simulink model "Lab13remix"  (R2025b)
settings: Solver=VariableStepAuto  StartTime=0.0  StopTime=30  RelTol=1e-3
values from neighbouring files (symbols this model uses):
  CDdatum = CD(1:47,2)    [Presimulink.m]
  CLdatum = CL(1:47,2)    [Presimulink.m]
  Cmdatum = Cm(1:47,2)    [Presimulink.m]
  dCDelev = [dCDn10 dCDn5 dCD0 dCDp5 dCDp10]    [Presimulink.m]
  dCLelev = [dCLn10 dCLn5 dCL0 dCLp5 dCLp10]    [Presimulink.m]
  dCmelev = [dCmn10 dCmn5 dCm0 dCmp5 dCmp10]    [Presimulink.m]
undefined symbols (not defined in the file or in its folder): Cn_datum, Croll_datum, CY_datum, dCn_aileron, dCn_rudder, dCroll_aileron, dCroll_rudder, dCY_aileron, dCY_rudder
libraries: aerolibadyn x1, aerolibasang x1, aerolibanim x1
settings Model: Creator=andyf  LastModifiedBy=andyf

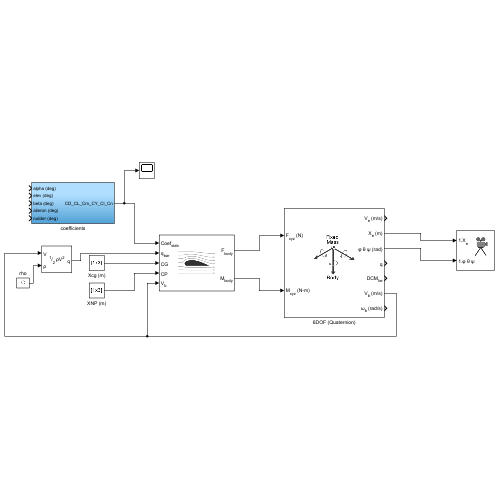
[thumbnail: Simulink's stored preview of the top-level diagram]
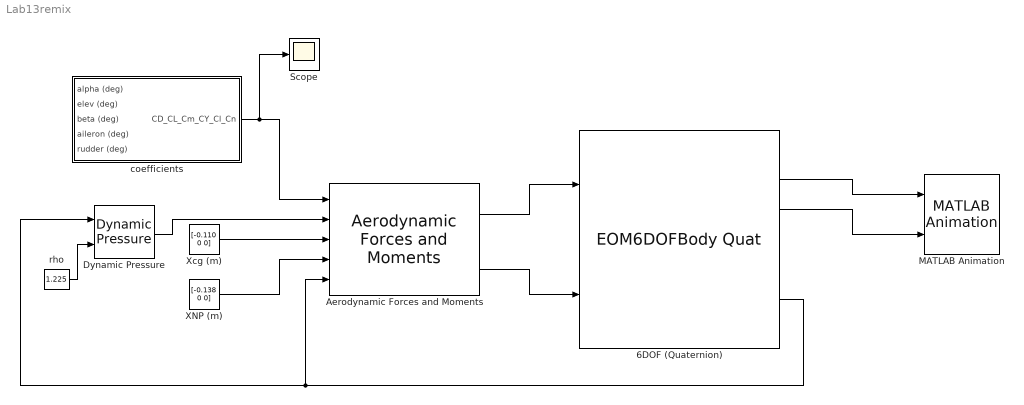
== system Lab13remix ==
  6DOF (Quaternion) : EOM6DOFBodyQuat  xme_0=[0 0 -200]  Vm_0=[15 0 2.5]  eul_0=[0 1.4*pi/180 0]  mass_0=0.45
  "Aerodynamic Forces and Moments " : aerolibadyn/Aerodynamic Forces and Moments   inputAxes=Stability  outputForceAxes=Body  outputMomentAxes=Body  S=0.15  b=1  cbar=0.156
  Dynamic Pressure : aerolibasang/Dynamic Pressure
  MATLAB Animation : aerolibanim/MATLAB Animation  Tag=Matlab Animation 6 DOF  Vehicles=1  Geometries='astredwedge.mat'  BoundingBoxCoordinates=[-50,50,-50,50,-50,50]  CameraOffset=[-150,-50,0]  CameraViewAngle=3  SampleTime=0.2  FigurePosition=[8.014000e+02,208,4.480000e+02,450]
  Scope : Scope
      settings: ActiveDisplayYMinimum=-0.18143250188090621  ActiveDisplayYMaximum=0.139826593948562
  XNP (m) : Constant  Value=[-0.138 0 0]
  Xcg (m) : Constant  Value=[-0.110 0 0]
  coefficients : Subsystem
  rho : Constant  Value=1.225
  wires:
  coefficients/1(CD_CL_Cm_CY_Cl_Cn) -> Scope/1, "Aerodynamic Forces and Moments "/1
  Xcg (m)/1 -> "Aerodynamic Forces and Moments "/3
  XNP (m)/1 -> "Aerodynamic Forces and Moments "/4
  "Aerodynamic Forces and Moments "/1 -> 6DOF (Quaternion)/1
  "Aerodynamic Forces and Moments "/2 -> 6DOF (Quaternion)/2
  rho/1 -> Dynamic Pressure/2
  6DOF (Quaternion)/6 -> Dynamic Pressure/1, "Aerodynamic Forces and Moments "/5
  Dynamic Pressure/1 -> "Aerodynamic Forces and Moments "/2
  6DOF (Quaternion)/3 -> MATLAB Animation/2
  6DOF (Quaternion)/2 -> MATLAB Animation/1

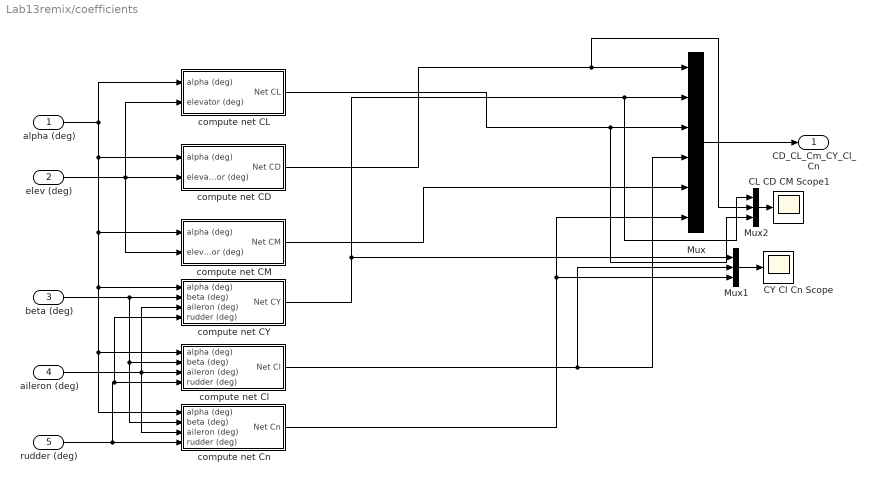
== system Lab13remix/coefficients ==
  alpha (deg) : Inport
  elev (deg) : Inport  Port=2
  beta (deg) : Inport  Port=3
  aileron (deg) : Inport  Port=4
  rudder (deg) : Inport  Port=5
  CL CD CM Scope1 : Scope
      settings: ActiveDisplayYMinimum=-5.92708  ActiveDisplayYMaximum=4.2418  DataLoggingVariableName=ScopeData4
  CY Cl Cn Scope : Scope
      settings: ActiveDisplayYMinimum=-0.00278  ActiveDisplayYMaximum=0.00326  DataLoggingVariableName=ScopeData3
  Mux : Mux  Inputs=6
  Mux1 : Mux  Inputs=3
  Mux2 : Mux  Inputs=3
  compute net CD : Subsystem
  compute net CL : Subsystem
  compute net CM : Subsystem
  compute net CY : Subsystem
  compute net Cl : Subsystem
  compute net Cn : Subsystem
  CD_CL_Cm_CY_Cl_Cn : Outport  VectorParamsAs1DForOutWhenUnconnected=off
  wires:
  compute net Cn/1(Net Cn) -> Mux1/3, Mux/6
  Mux/1 -> CD_CL_Cm_CY_Cl_Cn/1
  elev (deg)/1 -> compute net CD/2(elevator (deg)), compute net CM/2(elevator (deg)), compute net CL/2(elevator (deg))
  alpha (deg)/1 -> compute net CD/1(alpha (deg)), compute net Cn/1(alpha (deg)), compute net Cl/1(alpha (deg)), compute net CY/1(alpha (deg)), compute net CM/1(alpha (deg)), compute net CL/1(alpha (deg))
  compute net CD/1(Net CD) -> Mux2/2, Mux/1
  compute net CL/1(Net CL) -> Mux2/3, Mux/3
  compute net CM/1(Net CM) -> Mux/5
  compute net Cl/1(Net Cl) -> Mux1/2, Mux/4
  compute net CY/1(Net CY) -> Mux1/1, Mux2/1, Mux/2
  aileron (deg)/1 -> compute net Cl/3(aileron (deg)), compute net CY/3(aileron (deg)), compute net Cn/3(aileron (deg))
  beta (deg)/1 -> compute net Cn/2(beta (deg)), compute net Cl/2(beta (deg)), compute net CY/2(beta (deg))
  rudder (deg)/1 -> compute net CY/4(rudder (deg)), compute net Cl/4(rudder (deg)), compute net Cn/4(rudder (deg))
  Mux1/1 -> CY Cl Cn Scope/1
  Mux2/1 -> CL CD CM Scope1/1

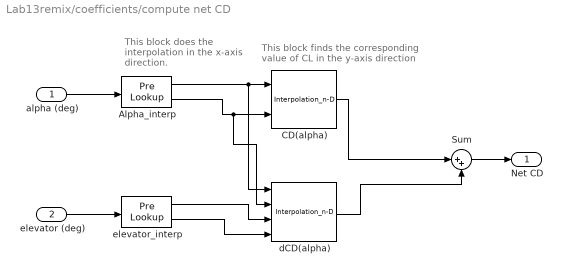
== system Lab13remix/coefficients/compute net CD ==
  note: This block finds the corresponding
      | value of CL in the y-axis direction
  note: This block does the interpolation in the
      | x-axis direction.
  alpha (deg) : Inport
  elevator (deg) : Inport  Port=2
  Alpha_interp : PreLookup  BreakpointsData=alpha  BeginIndexSearchUsingPreviousIndexResult=on  ExtrapMethod=Linear
  CD(alpha) : Interpolation_n-D  NumberOfTableDimensions=1  Table=CDdatum  RemoveProtectionIndex=on
      settings: InputPortMap=u0,u1
  Sum : Sum  Inputs=|++
  dCD(alpha) : Interpolation_n-D  Table=dCDelev
  elevator_interp : PreLookup  BreakpointsData=delev  BeginIndexSearchUsingPreviousIndexResult=on  ExtrapMethod=Linear
  Net CD : Outport  VectorParamsAs1DForOutWhenUnconnected=off
  wires:
  Alpha_interp/1 -> dCD(alpha)/1, CD(alpha)/1
  Alpha_interp/2 -> dCD(alpha)/2, CD(alpha)/2
  CD(alpha)/1 -> Sum/1
  alpha (deg)/1 -> Alpha_interp/1
  elevator (deg)/1 -> elevator_interp/1
  elevator_interp/2 -> dCD(alpha)/4
  elevator_interp/1 -> dCD(alpha)/3
  dCD(alpha)/1 -> Sum/2
  Sum/1 -> Net CD/1

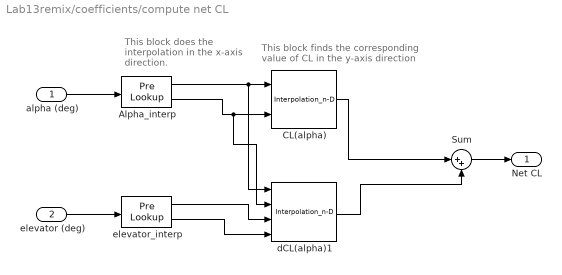
== system Lab13remix/coefficients/compute net CL ==
  note: This block finds the corresponding
      | value of CL in the y-axis direction
  note: This block does the interpolation in the
      | x-axis direction.
  alpha (deg) : Inport
  elevator (deg) : Inport  Port=2
  Alpha_interp : PreLookup  BreakpointsData=alpha  BeginIndexSearchUsingPreviousIndexResult=on  ExtrapMethod=Linear
  CL(alpha) : Interpolation_n-D  NumberOfTableDimensions=1  Table=CLdatum  RemoveProtectionIndex=on
      settings: InputPortMap=u0,u1
  Sum : Sum  Inputs=|++
  dCL(alpha)1 : Interpolation_n-D  Table=dCLelev
  elevator_interp : PreLookup  BreakpointsData=delev  BeginIndexSearchUsingPreviousIndexResult=on  ExtrapMethod=Linear
  Net CL : Outport  VectorParamsAs1DForOutWhenUnconnected=off
  wires:
  Alpha_interp/1 -> dCL(alpha)1/1, CL(alpha)/1
  Alpha_interp/2 -> dCL(alpha)1/2, CL(alpha)/2
  CL(alpha)/1 -> Sum/1
  alpha (deg)/1 -> Alpha_interp/1
  elevator (deg)/1 -> elevator_interp/1
  elevator_interp/2 -> dCL(alpha)1/4
  elevator_interp/1 -> dCL(alpha)1/3
  dCL(alpha)1/1 -> Sum/2
  Sum/1 -> Net CL/1

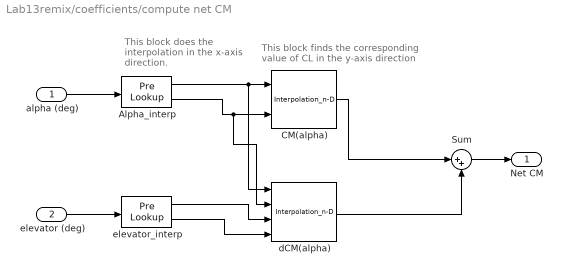
== system Lab13remix/coefficients/compute net CM ==
  note: This block finds the corresponding
      | value of CL in the y-axis direction
  note: This block does the interpolation in the
      | x-axis direction.
  alpha (deg) : Inport
  elevator (deg) : Inport  Port=2
  Alpha_interp : PreLookup  BreakpointsData=alpha  BeginIndexSearchUsingPreviousIndexResult=on  ExtrapMethod=Linear
  CM(alpha) : Interpolation_n-D  NumberOfTableDimensions=1  Table=Cmdatum  RemoveProtectionIndex=on
      settings: InputPortMap=u0,u1
  Sum : Sum  Inputs=|++
  dCM(alpha) : Interpolation_n-D  Table=dCmelev
  elevator_interp : PreLookup  BreakpointsData=delev  BeginIndexSearchUsingPreviousIndexResult=on  ExtrapMethod=Linear
  Net CM : Outport  VectorParamsAs1DForOutWhenUnconnected=off
  wires:
  Alpha_interp/1 -> dCM(alpha)/1, CM(alpha)/1
  Alpha_interp/2 -> dCM(alpha)/2, CM(alpha)/2
  CM(alpha)/1 -> Sum/1
  alpha (deg)/1 -> Alpha_interp/1
  elevator (deg)/1 -> elevator_interp/1
  elevator_interp/2 -> dCM(alpha)/4
  elevator_interp/1 -> dCM(alpha)/3
  Sum/1 -> Net CM/1
  dCM(alpha)/1 -> Sum/2

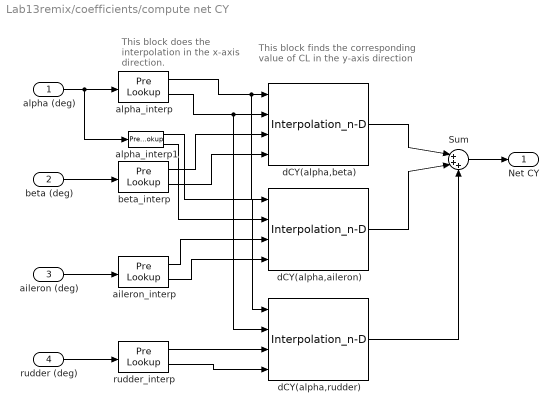
== system Lab13remix/coefficients/compute net CY ==
  note: This block finds the corresponding
      | value of CL in the y-axis direction
  note: This block does the interpolation in the
      | x-axis direction.
  alpha (deg) : Inport
  beta (deg) : Inport  Port=2
  aileron (deg) : Inport  Port=3
  rudder (deg) : Inport  Port=4
  Sum : Sum  Inputs=|+++
  aileron_interp : PreLookup  BreakpointsData=aileron  BeginIndexSearchUsingPreviousIndexResult=on  ExtrapMethod=Linear
  alpha_interp : PreLookup  BreakpointsData=alphalatrud  BeginIndexSearchUsingPreviousIndexResult=on  ExtrapMethod=Linear
  alpha_interp1 : PreLookup  BreakpointsData=alphaaileron  BeginIndexSearchUsingPreviousIndexResult=on  ExtrapMethod=Linear
  beta_interp : PreLookup  BreakpointsData=beta  BeginIndexSearchUsingPreviousIndexResult=on  ExtrapMethod=Linear
  dCY(alpha,aileron) : Interpolation_n-D  Table=dCY_aileron
  dCY(alpha,beta) : Interpolation_n-D  Table=CY_datum
  dCY(alpha,rudder) : Interpolation_n-D  Table=dCY_rudder
  rudder_interp : PreLookup  BreakpointsData=rudder  BeginIndexSearchUsingPreviousIndexResult=on  ExtrapMethod=Linear
  Net CY : Outport  VectorParamsAs1DForOutWhenUnconnected=off
  wires:
  beta (deg)/1 -> beta_interp/1
  Sum/1 -> Net CY/1
  aileron (deg)/1 -> aileron_interp/1
  rudder (deg)/1 -> rudder_interp/1
  beta_interp/1 -> dCY(alpha,beta)/3
  beta_interp/2 -> dCY(alpha,beta)/4
  rudder_interp/2 -> dCY(alpha,rudder)/4
  aileron_interp/1 -> dCY(alpha,aileron)/3
  aileron_interp/2 -> dCY(alpha,aileron)/4
  rudder_interp/1 -> dCY(alpha,rudder)/3
  alpha (deg)/1 -> alpha_interp1/1, alpha_interp/1
  alpha_interp/2 -> dCY(alpha,rudder)/2, dCY(alpha,beta)/2
  alpha_interp/1 -> dCY(alpha,rudder)/1, dCY(alpha,beta)/1
  dCY(alpha,aileron)/1 -> Sum/2
  dCY(alpha,beta)/1 -> Sum/1
  alpha_interp1/1 -> dCY(alpha,aileron)/1
  alpha_interp1/2 -> dCY(alpha,aileron)/2
  dCY(alpha,rudder)/1 -> Sum/3

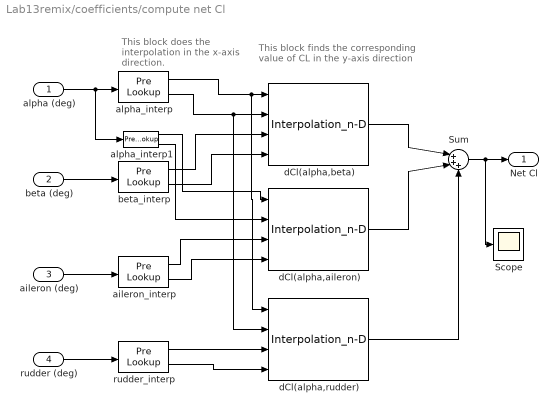
== system Lab13remix/coefficients/compute net Cl ==
  note: This block finds the corresponding
      | value of CL in the y-axis direction
  note: This block does the interpolation in the
      | x-axis direction.
  alpha (deg) : Inport
  beta (deg) : Inport  Port=2
  aileron (deg) : Inport  Port=3
  rudder (deg) : Inport  Port=4
  Scope : Scope
      settings: ActiveDisplayYMinimum=-6E-5  ActiveDisplayYMaximum=0.00127  DataLoggingVariableName=ScopeData2
  Sum : Sum  Inputs=|+++
  aileron_interp : PreLookup  BreakpointsData=aileron  BeginIndexSearchUsingPreviousIndexResult=on  ExtrapMethod=Linear
  alpha_interp : PreLookup  BreakpointsData=alphalatrud  BeginIndexSearchUsingPreviousIndexResult=on  ExtrapMethod=Linear
  alpha_interp1 : PreLookup  BreakpointsData=alphaaileron  BeginIndexSearchUsingPreviousIndexResult=on  ExtrapMethod=Linear
  beta_interp : PreLookup  BreakpointsData=beta  BeginIndexSearchUsingPreviousIndexResult=on  ExtrapMethod=Linear
  dCl(alpha,aileron) : Interpolation_n-D  Table=dCroll_aileron
  dCl(alpha,beta) : Interpolation_n-D  Table=Croll_datum
  dCl(alpha,rudder) : Interpolation_n-D  Table=dCroll_rudder
  rudder_interp : PreLookup  BreakpointsData=rudder  BeginIndexSearchUsingPreviousIndexResult=on  ExtrapMethod=Linear
  Net Cl : Outport  VectorParamsAs1DForOutWhenUnconnected=off
  wires:
  beta (deg)/1 -> beta_interp/1
  Sum/1 -> Scope/1, Net Cl/1
  aileron (deg)/1 -> aileron_interp/1
  rudder (deg)/1 -> rudder_interp/1
  beta_interp/1 -> dCl(alpha,beta)/3
  beta_interp/2 -> dCl(alpha,beta)/4
  rudder_interp/2 -> dCl(alpha,rudder)/4
  aileron_interp/1 -> dCl(alpha,aileron)/3
  aileron_interp/2 -> dCl(alpha,aileron)/4
  rudder_interp/1 -> dCl(alpha,rudder)/3
  alpha (deg)/1 -> alpha_interp1/1, alpha_interp/1
  alpha_interp/2 -> dCl(alpha,rudder)/2, dCl(alpha,beta)/2
  alpha_interp/1 -> dCl(alpha,rudder)/1, dCl(alpha,beta)/1
  dCl(alpha,aileron)/1 -> Sum/2
  dCl(alpha,rudder)/1 -> Sum/3
  dCl(alpha,beta)/1 -> Sum/1
  alpha_interp1/1 -> dCl(alpha,aileron)/1
  alpha_interp1/2 -> dCl(alpha,aileron)/2

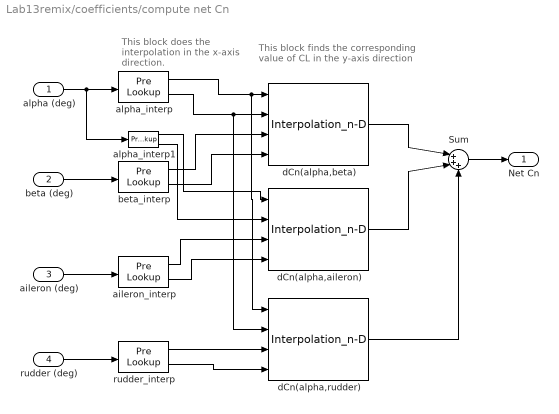
== system Lab13remix/coefficients/compute net Cn ==
  note: This block finds the corresponding
      | value of CL in the y-axis direction
  note: This block does the interpolation in the
      | x-axis direction.
  alpha (deg) : Inport
  beta (deg) : Inport  Port=2
  aileron (deg) : Inport  Port=3
  rudder (deg) : Inport  Port=4
  Sum : Sum  Inputs=|+++
  aileron_interp : PreLookup  BreakpointsData=aileron  BeginIndexSearchUsingPreviousIndexResult=on  ExtrapMethod=Linear
  alpha_interp : PreLookup  BreakpointsData=alphalatrud  BeginIndexSearchUsingPreviousIndexResult=on  ExtrapMethod=Linear
  alpha_interp1 : PreLookup  BreakpointsData=alphaaileron  BeginIndexSearchUsingPreviousIndexResult=on  ExtrapMethod=Linear
  beta_interp : PreLookup  BreakpointsData=beta  BeginIndexSearchUsingPreviousIndexResult=on  ExtrapMethod=Linear
  dCn(alpha,aileron) : Interpolation_n-D  Table=dCn_aileron
  dCn(alpha,beta) : Interpolation_n-D  Table=Cn_datum
  dCn(alpha,rudder) : Interpolation_n-D  Table=dCn_rudder
  rudder_interp : PreLookup  BreakpointsData=rudder  BeginIndexSearchUsingPreviousIndexResult=on  ExtrapMethod=Linear
  Net Cn : Outport  VectorParamsAs1DForOutWhenUnconnected=off
  wires:
  beta (deg)/1 -> beta_interp/1
  Sum/1 -> Net Cn/1
  aileron (deg)/1 -> aileron_interp/1
  rudder (deg)/1 -> rudder_interp/1
  beta_interp/1 -> dCn(alpha,beta)/3
  beta_interp/2 -> dCn(alpha,beta)/4
  rudder_interp/2 -> dCn(alpha,rudder)/4
  aileron_interp/1 -> dCn(alpha,aileron)/3
  aileron_interp/2 -> dCn(alpha,aileron)/4
  rudder_interp/1 -> dCn(alpha,rudder)/3
  alpha (deg)/1 -> alpha_interp1/1, alpha_interp/1
  alpha_interp/2 -> dCn(alpha,rudder)/2, dCn(alpha,beta)/2
  alpha_interp/1 -> dCn(alpha,rudder)/1, dCn(alpha,beta)/1
  dCn(alpha,beta)/1 -> Sum/1
  dCn(alpha,aileron)/1 -> Sum/2
  dCn(alpha,rudder)/1 -> Sum/3
  alpha_interp1/1 -> dCn(alpha,aileron)/1
  alpha_interp1/2 -> dCn(alpha,aileron)/2
